simulink model "StepperMotor2021"  (R2021b)
settings: Solver=VariableStepAuto  StartTime=0.0  StopTime=10.0  RelTol=1e-3
values from neighbouring files (symbols this model uses):
  a1 = Beq + (ng* Kg^2 * nm* Kt * Km/Rm)    (= 0.07285017685)    [Lab4.m]
  a2 = Jeq    (= 0.002)    [Lab4.m]
  b = ng*Kg*nm*Kt/Rm    (= 0.1282365)    [Lab4.m]
  Kd = (2*zeta*wn*a2 - a1)/b    [Lab4.m]
  Kp = Kp - 8.5    [Lab4.m]
settings Model: Creator=17165  LastModifiedBy=17165

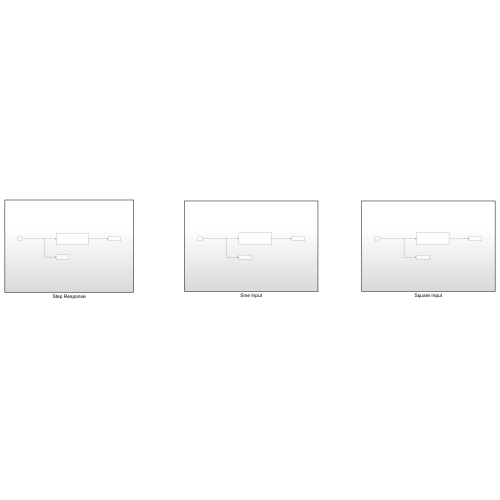
[thumbnail: Simulink's stored preview of the top-level diagram]
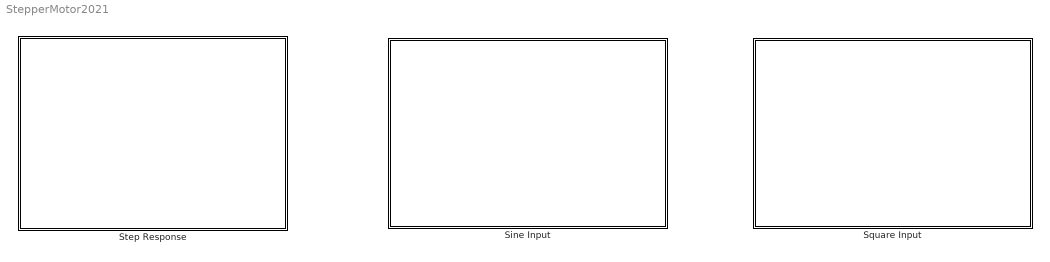
== system StepperMotor2021 ==
  Sine Input : Subsystem
  Square Input : Subsystem
  Step Response : Subsystem

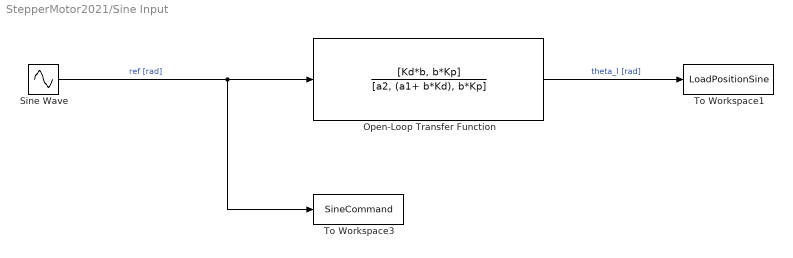
== system StepperMotor2021/Sine Input ==
  Open-Loop Transfer Function : TransferFcn  Numerator=[Kd*b, b*Kp]  Denominator=[a2, (a1+ b*Kd), b*Kp]
  Sine Wave : Sin  Frequency=5  SampleTime=0
  To Workspace1 : ToWorkspace  VariableName=LoadPositionSine  SampleTime=-1
  To Workspace3 : ToWorkspace  VariableName=SineCommand  SampleTime=-1
  wires:
  Sine Wave/1 -> To Workspace3/1, Open-Loop Transfer Function/1  "ref [rad]"
  Open-Loop Transfer Function/1 -> To Workspace1/1  "theta_l [rad]"

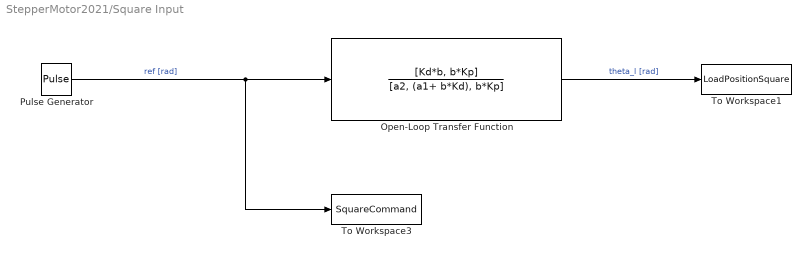
== system StepperMotor2021/Square Input ==
  Open-Loop Transfer Function : TransferFcn  Numerator=[Kd*b, b*Kp]  Denominator=[a2, (a1+ b*Kd), b*Kp]
  Pulse Generator : DiscretePulseGenerator  PulseType=Time based  Period=1  PulseWidth=50
  To Workspace1 : ToWorkspace  VariableName=LoadPositionSquare  SampleTime=-1
  To Workspace3 : ToWorkspace  VariableName=SquareCommand  SampleTime=-1
  wires:
  Pulse Generator/1 -> To Workspace3/1, Open-Loop Transfer Function/1  "ref [rad]"
  Open-Loop Transfer Function/1 -> To Workspace1/1  "theta_l [rad]"

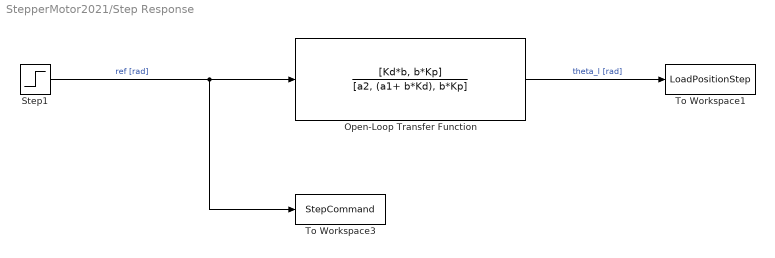
== system StepperMotor2021/Step Response ==
  Open-Loop Transfer Function : TransferFcn  Numerator=[Kd*b, b*Kp]  Denominator=[a2, (a1+ b*Kd), b*Kp]
  Step1 : Step  SampleTime=0
  To Workspace1 : ToWorkspace  VariableName=LoadPositionStep  SampleTime=-1
  To Workspace3 : ToWorkspace  VariableName=StepCommand  SampleTime=-1
  wires:
  Step1/1 -> To Workspace3/1, Open-Loop Transfer Function/1  "ref [rad]"
  Open-Loop Transfer Function/1 -> To Workspace1/1  "theta_l [rad]"
